simulink model "Res_22"  (R2013b)
settings: Solver=ode4  StartTime=0.0  StopTime=25  RelTol=1e-3
values from neighbouring files (symbols this model uses):
  A = [0 1 0 0 0 0 ... (first row only)    [result_22.m]
  B = [0;1/m1;0;0;0;0]    [result_22.m]
  C = [0 1 0 0 0 0 ... (first row only)    [result_22.m]
  D = [0;0]    [result_22.m]
settings Model: Creator=makha  LastModifiedBy=Zeerak Nadeem Wyne
settings DataIOCC: LimitDataPoints=off  SaveFormat=Dataset
settings OptimizationCC: LifeSpan=auto  SimCompilerOptimization=off
settings DebuggingCC: UnderspecifiedInitializationDetection=Simplified  MergeDetectMultiDrivingBlocksExec=error  SolverPrmCheckMsg=none  FcnCallInpInsideContextMsg=error  FrameProcessingCompatibilityMsg=error  LibraryContextMissingDiagnostic=warning  SFUnexpectedBacktrackingDiag=error  SFNoUnconditionalDefaultTransitionDiag=error
settings HardwareCC: ProdBitPerPointer=64  ProdLargestAtomicFloat=Float  ProdIntDivRoundTo=Zero  ProdEndianess=LittleEndian  ProdWordSize=64  ProdHWDeviceType=Intel->x86-64 (Windows64)
settings ModelReferenceCC: PropagateSignalLabelsOutOfModel=on
settings SFSimCC: SimUseLocalCustomCode=on
settings RTWCC: RTWUseLocalCustomCode=on  RTWCompilerOptimization=off
settings GRTTargetCC: CodeReplacementLibrary=None  GeneratePreprocessorConditionals=Use local settings  CPPClassGenCompliant=on

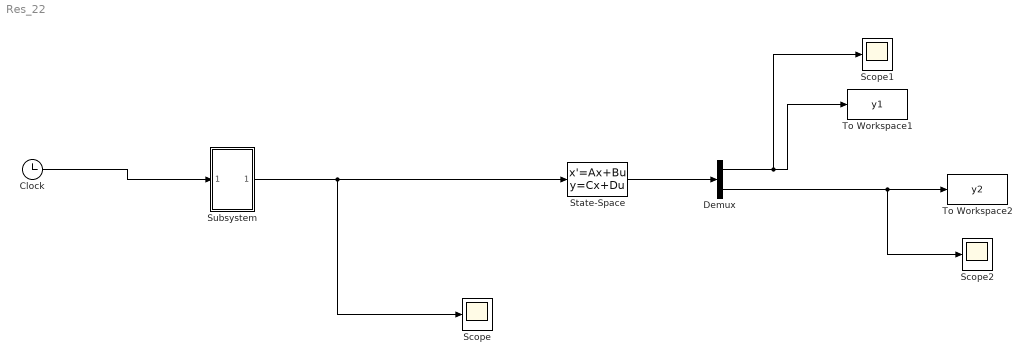
== system Res_22 ==
  Clock : Clock
      settings: Decimation=1000
  Demux : Demux  Outputs=2
  Scope : Scope
  Scope1 : Scope
  Scope2 : Scope
      settings: SaveName=ScopeData2
  State-Space : StateSpace  A=A  B=B  C=C  D=D
  Subsystem : Subsystem
  To Workspace1 : ToWorkspace  VariableName=y1  SampleTime=-1
  To Workspace2 : ToWorkspace  VariableName=y2  SampleTime=-1
  wires:
  Demux/1 -> Scope1/1, To Workspace1/1
  Demux/2 -> Scope2/1, To Workspace2/1
  State-Space/1 -> Demux/1
  Subsystem/1(Out1) -> State-Space/1, Scope/1
  Clock/1 -> Subsystem/1(In1)

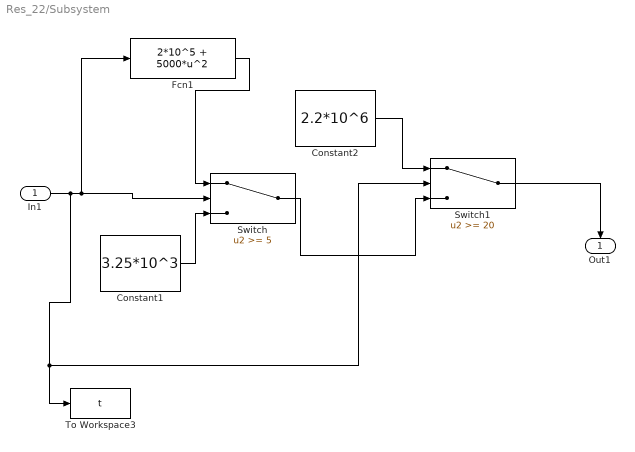
== system Res_22/Subsystem ==
  In1 : Inport
  Constant1 : Constant  Value=3.25*10^3
  Constant2 : Constant  Value=2.2*10^6
  Fcn1 : Fcn  Expr=2*10^5 + 5000*u^2
  Switch : Switch  Threshold=5  SaturateOnIntegerOverflow=off  InputSameDT=off
  Switch1 : Switch  Threshold=20  SaturateOnIntegerOverflow=off  InputSameDT=off
  To Workspace3 : ToWorkspace  VariableName=t  SampleTime=-1
  Out1 : Outport
  wires:
  In1/1 -> Switch1/2, To Workspace3/1, Fcn1/1, Switch/2
  Switch/1 -> Switch1/3
  Constant1/1 -> Switch/3
  Switch1/1 -> Out1/1
  Fcn1/1 -> Switch/1
  Constant2/1 -> Switch1/1
